simulink model "demosignal"  (R2023b)
settings: Solver=VariableStepAuto  StartTime=0.0  StopTime=0.005  RelTol=1e-3
libraries: eeGeneralControl x2
settings Model: Creator=Tonda  LastModifiedBy=Tonda

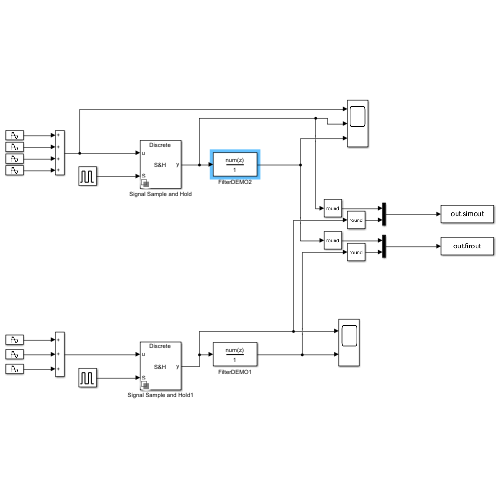
[thumbnail: Simulink's stored preview of the top-level diagram]
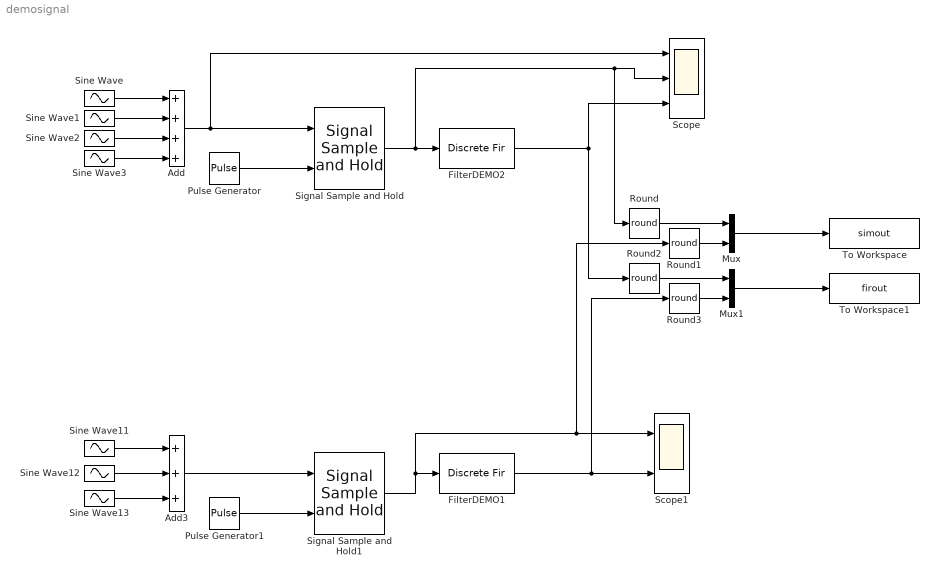
== system demosignal ==
  Add : Sum  Inputs=++++
  Add3 : Sum  Inputs=+++
  FilterDEMO1 : DiscreteFir  Tag=BlockMethodSubSystem  Coefficients=[0 -0.000379417487354319393 -0.000731741696903727814 0.0044427097150600732 0.0104146029900219188 -0.0103473390201568698 -0.0510778424546868351 -0.0124939820877546948 0.177073771908299538 0.383099238133474962 0.383099238133474962 0.177073771908299538 -0.0124939820877546948 -0.0510778424546868351 -0.0103473390201568698 0.0104146029900219188 0.0044427097150600732 -0.000731741696903727814 -0.000379417487354319393 0]  InputProcessing=Columns as channels (frame based)
  FilterDEMO2 : DiscreteFir  Tag=BlockMethodSubSystem  Coefficients=[0 -0.000379417487354319393 -0.000731741696903727814 0.0044427097150600732 0.0104146029900219188 -0.0103473390201568698 -0.0510778424546868351 -0.0124939820877546948 0.177073771908299538 0.383099238133474962 0.383099238133474962 0.177073771908299538 -0.0124939820877546948 -0.0510778424546868351 -0.0103473390201568698 0.0104146029900219188 0.0044427097150600732 -0.000731741696903727814 -0.000379417487354319393 0]  InputProcessing=Columns as channels (frame based)
  Mux : Mux  Inputs=2
  Mux1 : Mux  Inputs=2
  Pulse Generator : DiscretePulseGenerator  PulseType=Time based  Period=1/48000
  Pulse Generator1 : DiscretePulseGenerator  PulseType=Time based  Period=1/48000
  Round{,1..3} (4 alike) : Rounding  Operator=round
  Scope : Scope  NumInputPorts=3
  Scope1 : Scope  NumInputPorts=2
  Signal Sample and Hold : eeGeneralControl/Signal Sample and Hold  LabelModeActiveChoice=Discrete  x0=0  Ts=1/48000
      settings: LibrarySourceBlock=ee_sl_lib/General Control/Signal Sample and Hold
  Signal Sample and Hold1 : eeGeneralControl/Signal Sample and Hold  LabelModeActiveChoice=Discrete  x0=0  Ts=1/48000
      settings: LibrarySourceBlock=ee_sl_lib/General Control/Signal Sample and Hold
  Sine Wave : Sin  Amplitude=8000  Frequency=2*pi*1000  SampleTime=0
  Sine Wave1 : Sin  Amplitude=8000  Frequency=2*pi*8000  SampleTime=0
  Sine Wave11 : Sin  Amplitude=8000  Frequency=2*pi*500  SampleTime=0
  Sine Wave12 : Sin  Amplitude=8000  Frequency=2*pi*15000  SampleTime=0
  Sine Wave13 : Sin  Amplitude=8000  Frequency=2*pi*16000  SampleTime=0
  Sine Wave2 : Sin  Amplitude=8000  Frequency=2*pi*15000  SampleTime=0
  Sine Wave3 : Sin  Amplitude=8000  Frequency=2*pi*19000  SampleTime=0
  To Workspace : ToWorkspace  VariableName=simout  SampleTime=-1
  To Workspace1 : ToWorkspace  VariableName=firout  SampleTime=-1
  wires:
  Sine Wave/1 -> Add/1
  Sine Wave2/1 -> Add/3
  Sine Wave3/1 -> Add/4
  Sine Wave1/1 -> Add/2
  Pulse Generator/1 -> Signal Sample and Hold/2
  Add/1 -> Scope/1, Signal Sample and Hold/1
  FilterDEMO2/1 -> Round2/1, Scope/3
  FilterDEMO1/1 -> Round3/1, Scope1/2
  Add3/1 -> Signal Sample and Hold1/1
  Sine Wave11/1 -> Add3/1
  Sine Wave12/1 -> Add3/2
  Sine Wave13/1 -> Add3/3
  Signal Sample and Hold1/1 -> FilterDEMO1/1, Round1/1, Scope1/1
  Pulse Generator1/1 -> Signal Sample and Hold1/2
  Mux/1 -> To Workspace/1
  Mux1/1 -> To Workspace1/1
  Signal Sample and Hold/1 -> FilterDEMO2/1, Round/1, Scope/2
  Round/1 -> Mux/1
  Round1/1 -> Mux/2
  Round2/1 -> Mux1/1
  Round3/1 -> Mux1/2
